simulink model "Symmetric"  (R2025a)
settings: Solver=VariableStepAuto  StartTime=0.0  StopTime=10.0  RelTol=1e-3
libraries: spsDiodeLib x3, spsCurrentMeasurementLib x2, spsIGBTLib x2, spsVoltageMeasurementLib x2, spsACVoltageSourceLib x1, spsDCMachineLib x1, spsDCVoltageSourceLib x1, sps_lib x1
settings Model: Creator=aditl  LastModifiedBy=aditl
settings DataIOCC: ReturnWorkspaceOutputs=off

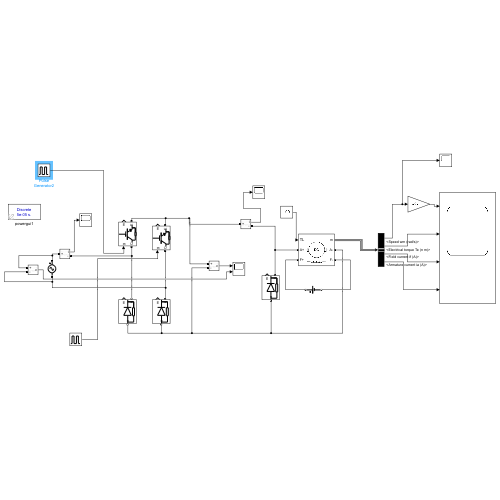
[thumbnail: Simulink's stored preview of the top-level diagram]
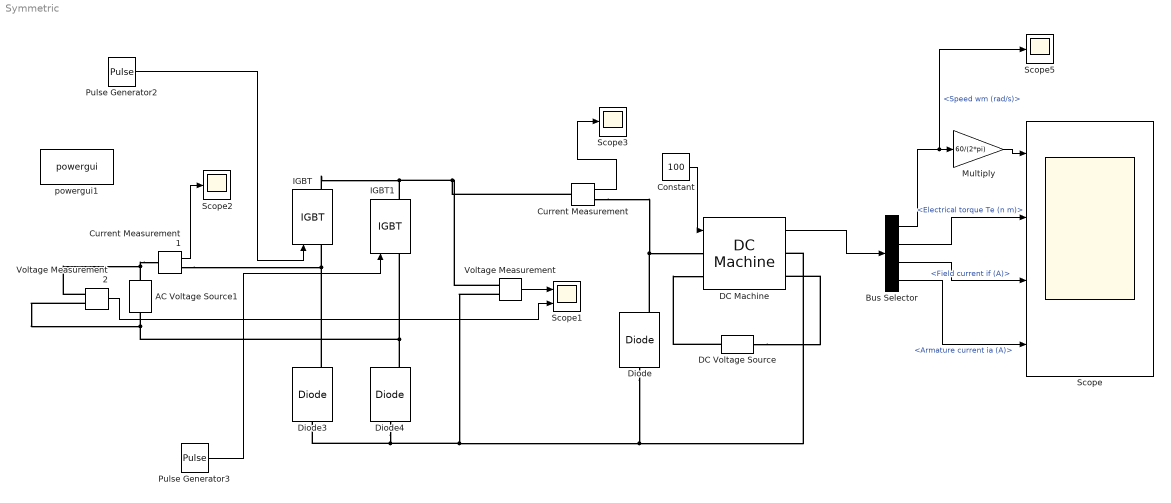
== system Symmetric ==
  AC Voltage Source1 : spsACVoltageSourceLib/AC Voltage Source  Amplitude=240*sqrt(2)  Phase=0  Frequency=50  SampleTime=0  Measurements=None  BusType=swing  Pref=10e3  Qref=0  Qmin=-inf  Qmax=+inf
  Bus Selector : BusSelector  OutputSignals=Speed wm (rad/s),Electrical torque Te (n m),Field current if (A),Armature current ia (A)
  Constant : Constant  Value=100
  Current Measurement : spsCurrentMeasurementLib/Current Measurement  PhasorSimulation=off  OutputType=Complex  PSBequivalent=0
  Current Measurement1 : spsCurrentMeasurementLib/Current Measurement  PhasorSimulation=off  OutputType=Complex  PSBequivalent=0
  DC Machine : spsDCMachineLib/DC Machine  PresetModel=02: 5HP 240V 1750RPM Field:150V  MechanicalLoad=Torque TL  FieldType=Wound  ShowDetailedParameters=on  MeasurementBus=off  RLa=[0.78 0.016]  RLf=[150 112.5]  Laf=1.234  MachineConstant=Torque constant (N.m/A)  Ke=1.8  Kt=1.8  J=0.05  Bm=0.01  Tf=0  w0=1  Ifinit=1  TsPowergui=0  TsBlock=-1
  DC Voltage Source : spsDCVoltageSourceLib/DC Voltage Source  Amplitude=150  Measurements=None
  Diode : spsDiodeLib/Diode  Ron=0.001  Lon=0  Vf=0.8  IC=0  UseSnubber=0  Rs=500  Cs=250e-9  Measurements=on
  Diode3 : spsDiodeLib/Diode  Ron=0.001  Lon=0  Vf=0.8  IC=0  UseSnubber=0  Rs=500  Cs=250e-9  Measurements=on
  Diode4 : spsDiodeLib/Diode  Ron=0.001  Lon=0  Vf=0.8  IC=0  UseSnubber=0  Rs=500  Cs=250e-9  Measurements=on
  IGBT : spsIGBTLib/IGBT  Ron=0.001  Lon=0  Vf=1  Tf=1e-6  Tt=2e-6  IC=0  Rs=1e5  Cs=inf  Measurements=on
  IGBT1 : spsIGBTLib/IGBT  Ron=0.001  Lon=0  Vf=1  Tf=1e-6  Tt=2e-6  IC=0  Rs=1e5  Cs=inf  Measurements=on
  Multiply : Gain  Gain=60/(2*pi)
  Pulse Generator2 : DiscretePulseGenerator  PulseType=Time based  Period=0.02  PulseWidth=((180-60)/360)*100  PhaseDelay=0.0016667  VectorParams1D=off
  Pulse Generator3 : DiscretePulseGenerator  PulseType=Time based  Period=0.02  PulseWidth=((180-60)/360)*100  PhaseDelay=0.011667
  Scope : Scope  NumInputPorts=4
      settings: ActiveDisplayYMinimum=-211.50421178097452  ActiveDisplayYMaximum=1290.407696454816
  Scope1 : Scope  NumInputPorts=2
      settings: ActiveDisplayYMinimum=-43.311335976924994  ActiveDisplayYMaximum=379.7969570851846
  Scope2 : Scope
      settings: DataLoggingVariableName=SourceCurrent
  Scope3 : Scope
      settings: DataLoggingVariableName=LoadCurrent
  Scope5 : Scope
      settings: ActiveDisplayYMinimum=-25.810675934675746  ActiveDisplayYMaximum=242.29599932913663  DataLoggingVariableName=ScopeData5
  Voltage Measurement : spsVoltageMeasurementLib/Voltage Measurement  PhasorSimulation=off  OutputType=Complex  PSBequivalent=0
  Voltage Measurement2 : spsVoltageMeasurementLib/Voltage Measurement  PhasorSimulation=off  OutputType=Complex  PSBequivalent=0
  powergui1 : sps_lib/powergui  Priority=1  SimulationMode=Discrete  SampleTime=50e-6  frequency=60  Iterations=50  frequencyindice=50  Pbase=100e6  ErrMax=1e-4  UnitsV=kV  UnitsW=MW  buscounter=0  FunctionMessages=off  echomessages=off  EnableUseOfTLC=off  CurrentSourceSwitches=off  DisableSnubberDevices=off  DisableRonSwitches=off  DisableVfSwitches=off  DisplayEquations=off  AutomaticDiscreteSolvers=off  SolverType=Tustin/Backward Euler (TBE)  Interpol=off  ExternalGateDelay=off  methode=off  Ts=100  x0status=blocks  SPID=on  SwTol=0  HookPort=off  NonlinearTolerance=1e-4  nMaxIteration=100  ContinueOnMaxIteration=off  RestoreLinks=warning  ResistiveCurrentMeasurement=off  Frange=[0:2:500]  Ylog=off  Xlog=on  ShowGrid=off  save=off  variable=ZData  structure=0  ZoomFFT=off  StartTime=0.0  cycles=1  DisplayStyle=1  fundamental=60  FreqAxis=off  MaxFrequency=1000  frequencyindicesteady=1  RmsSteady=1  display=off
  wires:
  Bus Selector/2 -> Scope/2  "<Electrical torque Te (n m)>"
  Pulse Generator3/1 -> IGBT1/1
  Bus Selector/3 -> Scope/3  "<Field current if (A)>"
  Voltage Measurement/1 -> Scope1/1
  Bus Selector/4 -> Scope/4  "<Armature current ia (A)>"
  Current Measurement1/1 -> Scope2/1
  Voltage Measurement2/1 -> Scope1/2
  Multiply/1 -> Scope/1
  Pulse Generator2/1 -> IGBT/1
  DC Machine/1 -> Bus Selector/1
  Current Measurement/1 -> Scope3/1
  Bus Selector/1 -> Scope5/1, Multiply/1  "<Speed wm (rad/s)>"
  Constant/1 -> DC Machine/1
  connections:
  Voltage Measurement2/LConn2 -- AC Voltage Source1/LConn1 -- Diode4/RConn1 -- IGBT1/LConn1
  Voltage Measurement/LConn2 -- Diode4/LConn1 -- Diode3/LConn1 -- Diode/LConn1 -- DC Machine/RConn1
  Diode/RConn1 -- Current Measurement/RConn1 -- DC Machine/LConn1
  IGBT/RConn1 -- Voltage Measurement/LConn1 -- Current Measurement/LConn1 -- IGBT1/RConn1
  Diode3/RConn1 -- IGBT/LConn1 -- Current Measurement1/RConn1
  Current Measurement1/LConn1 -- Voltage Measurement2/LConn1 -- AC Voltage Source1/RConn1
  DC Voltage Source/LConn1 -- DC Machine/RConn2
  DC Voltage Source/RConn1 -- DC Machine/LConn2
